simulink model "question_2_2"  (Simulink 8.8)
settings: Solver=FixedStepAuto  StartTime=0.0  StopTime=pi*8  FixedStep=0.01  RelTol=1e-3
libraries: simulink x2, fuzblock x2
settings Model: Creator=Dreamer  LastModifiedBy=Dreamer
settings DataIOCC: LimitDataPoints=off  SaveFormat=Dataset  SignalLoggingSaveFormat=Dataset
settings OptimizationCC: LifeSpan=auto
settings DebuggingCC: UnderspecifiedInitializationDetection=Simplified  MergeDetectMultiDrivingBlocksExec=error  FcnCallInpInsideContextMsg=error  StateNameClashWarn=none  SFUnexpectedBacktrackingDiag=error  SFNoUnconditionalDefaultTransitionDiag=error  SFExecutionAtInitializationDiag=warning
settings HardwareCC: ProdBitPerPointer=64  ProdBitPerSizeT=64  ProdBitPerPtrDiffT=64  ProdLargestAtomicFloat=Float  ProdIntDivRoundTo=Zero  ProdEndianess=LittleEndian  ProdWordSize=64  ProdHWDeviceType=Intel->x86-64 (Windows64)
settings ModelReferenceCC: PropagateSignalLabelsOutOfModel=on
settings GRTTargetCC: TargetLangStandard=C99 (ISO)  GeneratePreprocessorConditionals=Use local settings  CombineOutputUpdateFcns=on  GRTInterface=off
settings ConfigComp: CovMetricSettings=dwe  CovHtmlReporting=off  CovSaveCumulativeToWorkspaceVar=off  CovSaveSingleToWorkspaceVar=off  CovExternalEMLEnable=on

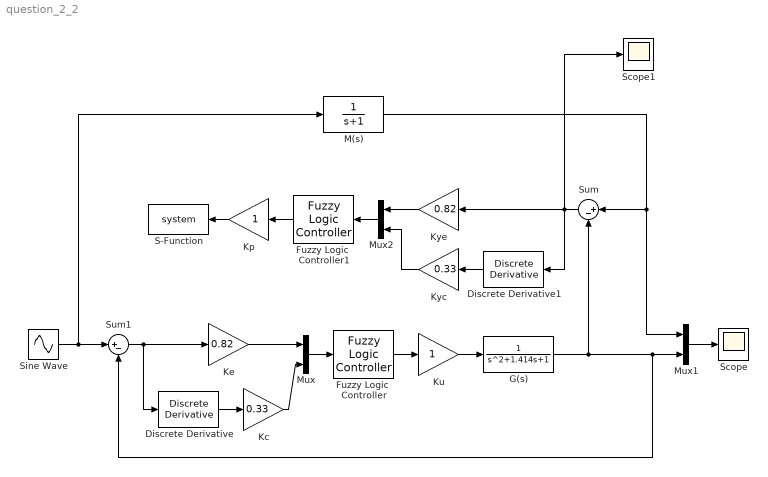
== system question_2_2 ==
  Discrete Derivative : simulink/Discrete/Discrete Derivative  gainval=1.0  ICPrevScaledInput=0.0  OutMin=[]  OutMax=[]  OutDataType=fixdt(1, 16)  OutScaling=2^-10  DoSatur=off
  Discrete Derivative1 : simulink/Discrete/Discrete Derivative  gainval=1.0  ICPrevScaledInput=0.0  OutMin=[]  OutMax=[]  OutDataType=fixdt(1, 16)  OutScaling=2^-10  DoSatur=off
  Fuzzy Logic  Controller : fuzblock/Fuzzy Logic  Controller  fis='question1.fis'
  Fuzzy Logic  Controller1 : fuzblock/Fuzzy Logic  Controller  fis='question1.fis'
  G(s) : TransferFcn  Denominator=[1 1.414 1]
  Kc : Gain  Gain=0.33
  Ke : Gain  Gain=0.82
  Kp : Gain
  Ku : Gain
  Kyc : Gain  Gain=0.33
  Kye : Gain  Gain=0.82
  M(s) : TransferFcn  Denominator=[1 1]
  Mux : Mux  Inputs=2
  Mux1 : Mux  Inputs=2
  Mux2 : Mux  Inputs=2
  S-Function : S-Function  SFunctionDeploymentMode=off  EnableBusSupport=off
  Scope : Scope
  Scope1 : Scope
  Sine Wave : Sin  Frequency=0.5  SampleTime=0
  Sum : Sum  Inputs=|+-
  Sum1 : Sum  Inputs=|+-
  wires:
  Ke/1 -> Mux/1
  Kc/1 -> Mux/2
  Mux/1 -> Fuzzy Logic  Controller/1
  Fuzzy Logic  Controller/1 -> Ku/1
  Ku/1 -> G(s)/1
  Mux1/1 -> Scope/1
  G(s)/1 -> Mux1/2, Sum1/2, Sum/2
  M(s)/1 -> Mux1/1, Sum/1
  Discrete Derivative/1 -> Kc/1
  Sum1/1 -> Discrete Derivative/1, Ke/1
  Sine Wave/1 -> M(s)/1, Sum1/1
  Sum/1 -> Discrete Derivative1/1, Kye/1, Scope1/1
  Discrete Derivative1/1 -> Kyc/1
  Kye/1 -> Mux2/1
  Kyc/1 -> Mux2/2
  Mux2/1 -> Fuzzy Logic  Controller1/1
  Fuzzy Logic  Controller1/1 -> Kp/1
  Kp/1 -> S-Function/1
